simulink model "Eq8to12_RC_Components"  (R2022b)
settings: Solver=VariableStepAuto  StartTime=0.0  StopTime=10.0  RelTol=1e-3
settings Model: Creator=umber  LastModifiedBy=umber
settings ModelReferenceCC: EnableRefExpFcnMdlSchedulingChecks=on

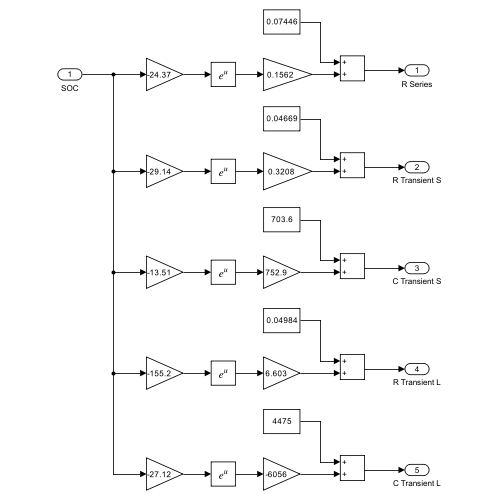
[thumbnail: Simulink's stored preview of the top-level diagram]
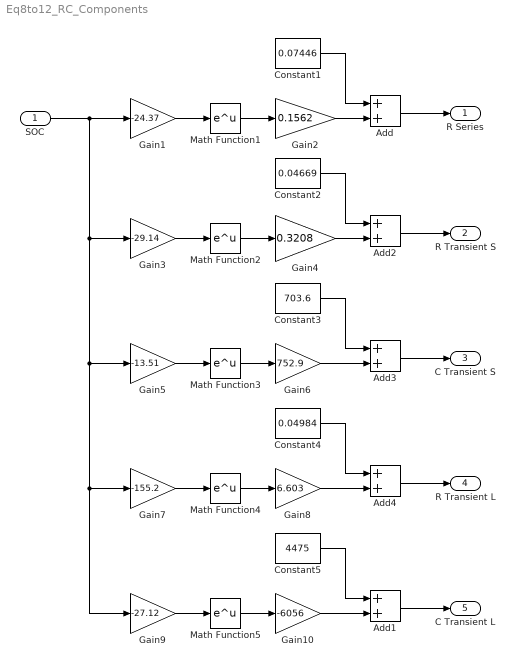
== system Eq8to12_RC_Components ==
  SOC : Inport
  Add{,1..4} (5 alike) : Sum
  Constant1 : Constant  Value=0.07446
  Constant2 : Constant  Value=0.04669
  Constant3 : Constant  Value=703.6
  Constant4 : Constant  Value=0.04984
  Constant5 : Constant  Value=4475
  Gain1 : Gain  Gain=-24.37
  Gain10 : Gain  Gain=-6056
  Gain2 : Gain  Gain=0.1562
  Gain3 : Gain  Gain=-29.14
  Gain4 : Gain  Gain=0.3208
  Gain5 : Gain  Gain=-13.51
  Gain6 : Gain  Gain=752.9
  Gain7 : Gain  Gain=-155.2
  Gain8 : Gain  Gain=6.603
  Gain9 : Gain  Gain=-27.12
  Math Function{1..5} (5 alike) : Math
  R Series : Outport
  R Transient S : Outport  Port=2
  C Transient S : Outport  Port=3
  R Transient L : Outport  Port=4
  C Transient L : Outport  Port=5
  wires:
  Gain2/1 -> Add/2
  Constant1/1 -> Add/1
  Math Function1/1 -> Gain2/1
  Gain1/1 -> Math Function1/1
  Add/1 -> R Series/1
  Gain4/1 -> Add2/2
  Add2/1 -> R Transient S/1
  Gain3/1 -> Math Function2/1
  Math Function2/1 -> Gain4/1
  Constant2/1 -> Add2/1
  Gain6/1 -> Add3/2
  Add3/1 -> C Transient S/1
  Gain5/1 -> Math Function3/1
  Math Function3/1 -> Gain6/1
  Constant3/1 -> Add3/1
  Gain8/1 -> Add4/2
  Add4/1 -> R Transient L/1
  Gain7/1 -> Math Function4/1
  Math Function4/1 -> Gain8/1
  Constant4/1 -> Add4/1
  Gain10/1 -> Add1/2
  SOC/1 -> Gain9/1, Gain7/1, Gain5/1, Gain3/1, Gain1/1
  Add1/1 -> C Transient L/1
  Gain9/1 -> Math Function5/1
  Math Function5/1 -> Gain10/1
  Constant5/1 -> Add1/1
